simulink model "example1"  (Simulink 8.7)
settings: Solver=ode45  StartTime=0.0  StopTime=10.0  MaxStep=0.2  RelTol=1e-3
undefined symbols (not defined in the file): FDab, planar
libraries: simulink x5
settings Model: Creator=roy  LastModifiedBy=Yaoting
settings DataIOCC: LimitDataPoints=off  SignalLoggingSaveFormat=ModelDataLogs
settings OptimizationCC: ExpressionDepthLimit=2147483647  InitFltsAndDblsToZero=on
settings DebuggingCC: SolverPrmCheckMsg=warning  FcnCallInpInsideContextMsg=UseLocalSettings  StateNameClashWarn=warning
settings GRTTargetCC: GeneratePreprocessorConditionals=Use local settings  CombineOutputUpdateFcns=off  GRTInterface=on

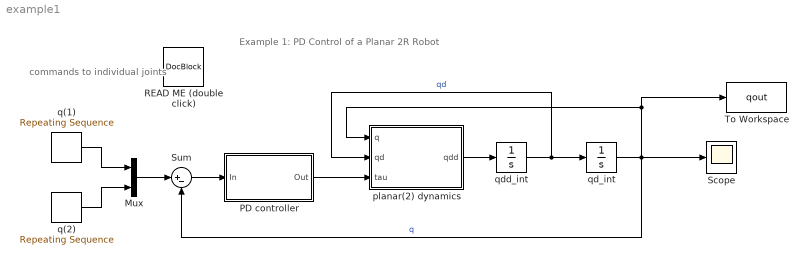
== system example1 ==
  note: Example 1: PD Control of a Planar 2R Robot
  note: commands to
      | individual
      | joints
  Mux : Mux  Inputs=2
  PD controller : Subsystem
  READ ME (double click) : simulink/Model-Wide Utilities/DocBlock  DocumentType=Text
  Scope : Scope
  Sum : Sum  Inputs=|+-
  To Workspace : ToWorkspace  VariableName=qout  SampleTime=-1
  planar(2) dynamics : Subsystem
  q(1) : simulink/Sources/Repeating Sequence  rep_seq_t=[0 1 2 3 4]  rep_seq_y=[0 1 1 0 0]
  q(2) : simulink/Sources/Repeating Sequence  rep_seq_t=[0 1 2 3 4]  rep_seq_y=[0 2 2 0 0]
  qd_int : Integrator
  qdd_int : Integrator
  wires:
  q(1)/1 -> Mux/1
  q(2)/1 -> Mux/2
  Mux/1 -> Sum/1
  Sum/1 -> PD controller/1(In)
  PD controller/1(Out) -> planar(2) dynamics/3(tau)
  planar(2) dynamics/1(qdd) -> qdd_int/1
  qdd_int/1 -> qd_int/1, planar(2) dynamics/2(qd)  "qd"
  qd_int/1 -> Scope/1, Sum/2, planar(2) dynamics/1(q), To Workspace/1  "q"

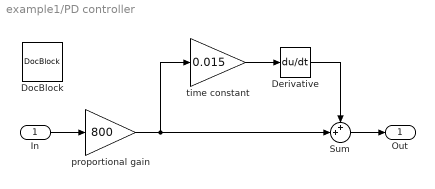
== system example1/PD controller ==
  In : Inport
  Derivative : Derivative
  DocBlock : simulink/Model-Wide Utilities/DocBlock  DocumentType=Text
  Sum : Sum  Inputs=++|
  proportional gain : Gain  Gain=800
  time constant : Gain  Gain=0.015
  Out : Outport
  wires:
  In/1 -> proportional gain/1
  proportional gain/1 -> Sum/2, time constant/1
  time constant/1 -> Derivative/1
  Derivative/1 -> Sum/1
  Sum/1 -> Out/1

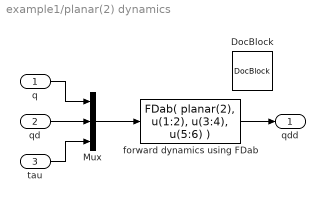
== system example1/planar(2) dynamics ==
  q : Inport
  qd : Inport  Port=2
  tau : Inport  Port=3
  DocBlock : simulink/Model-Wide Utilities/DocBlock  DocumentType=Text
  Mux : Mux  Inputs=3
  forward dynamics using FDab : MATLABFcn  MATLABFcn=FDab( planar(2), u(1:2), u(3:4), u(5:6) )  OutputDimensions=[2 1]  OutputSignalType=real  Output1D=off
  qdd : Outport
  wires:
  qd/1 -> Mux/2
  q/1 -> Mux/1
  tau/1 -> Mux/3
  Mux/1 -> forward dynamics using FDab/1
  forward dynamics using FDab/1 -> qdd/1
